simulink model "Controlador"  (R2023a)
settings: Solver=VariableStepAuto  StartTime=0.0  StopTime=60  RelTol=1e-3
values from neighbouring files (symbols this model uses):
  A = pi*R^2    (= 16971.6689129)    [Aerogerador.m]
  b = 46e3    (= 46000)    [Aerogerador.m]
  Cpmax0 = Cpmax(:, 1)    [Aerogerador.m]
  Ea_nom = Pnom/ia_nom    [Aerogerador.m]
  ia_nom = x(2, :)    [Aerogerador.m]
  J = 9e6    (= 9000000)    [Aerogerador.m]
  kv = 900*2    (= 1800)    [Aerogerador.m]
  La = 108e-3    (= 0.108)    [Aerogerador.m]
  lambdaopt = 7.5    [Aerogerador.m]    (also in funNominal.m)
  Ra = 100e-3    (= 0.1)    [Aerogerador.m]
  rho = 1.2    [Aerogerador.m]
  U_nom = x(1, :)    [Aerogerador.m]
  w_nom = (U_nom*lambdaopt)/R    [Aerogerador.m]
libraries: slpidlib x4
settings Model: Creator=danil  LastModifiedBy=danil

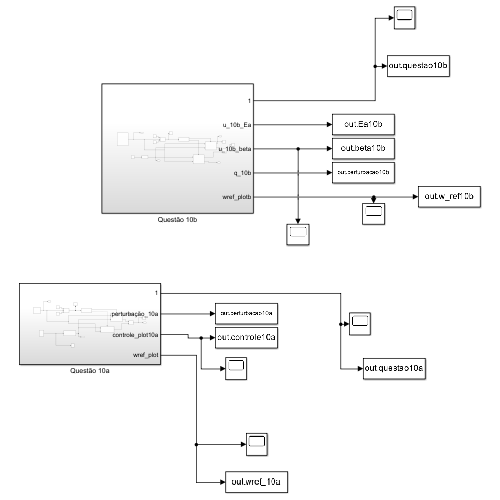
[thumbnail: Simulink's stored preview of the top-level diagram]
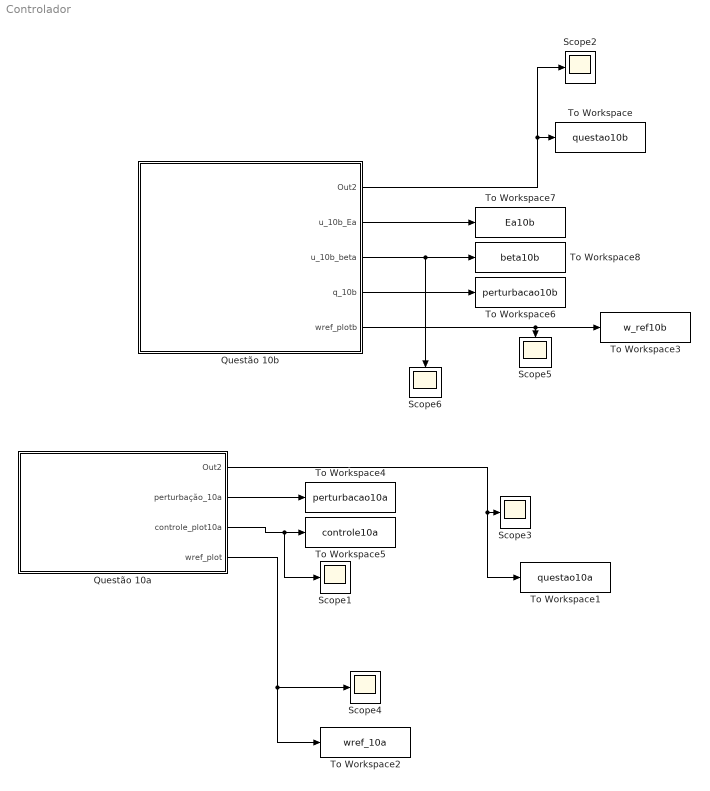
== system Controlador ==
  Questão 10a : Subsystem
  Questão 10b : Subsystem
  Scope{1..6} (6 alike) : Scope
  To Workspace : ToWorkspace  VariableName=questao10b  SampleTime=-1
      settings: Save2DSignal=2-D array (concatenate along first dimension)
  To Workspace1 : ToWorkspace  VariableName=questao10a  SampleTime=-1
      settings: Save2DSignal=2-D array (concatenate along first dimension)
  To Workspace2 : ToWorkspace  VariableName=wref_10a  SampleTime=-1
      settings: Save2DSignal=2-D array (concatenate along first dimension)
  To Workspace3 : ToWorkspace  VariableName=w_ref10b  SampleTime=-1
      settings: Save2DSignal=2-D array (concatenate along first dimension)
  To Workspace4 : ToWorkspace  VariableName=perturbacao10a  SampleTime=-1
      settings: Save2DSignal=2-D array (concatenate along first dimension)
  To Workspace5 : ToWorkspace  VariableName=controle10a  SampleTime=-1
      settings: Save2DSignal=2-D array (concatenate along first dimension)
  To Workspace6 : ToWorkspace  VariableName=perturbacao10b  SampleTime=-1
      settings: Save2DSignal=2-D array (concatenate along first dimension)
  To Workspace7 : ToWorkspace  VariableName=Ea10b  SampleTime=-1
      settings: Save2DSignal=2-D array (concatenate along first dimension)
  To Workspace8 : ToWorkspace  VariableName=beta10b  SampleTime=-1
      settings: Save2DSignal=2-D array (concatenate along first dimension)
  wires:
  Questão 10b/1(Out2) -> Scope2/1, To Workspace/1
  Questão 10a/1(Out2) -> To Workspace1/1, Scope3/1
  Questão 10a/4(wref_plot) -> To Workspace2/1, Scope4/1
  Questão 10b/5(wref_plotb) -> To Workspace3/1, Scope5/1
  Questão 10a/3(controle_plot10a) -> Scope1/1, To Workspace5/1
  Questão 10a/2(perturbação_10a) -> To Workspace4/1
  Questão 10b/4(q_10b) -> To Workspace6/1
  Questão 10b/2(u_10b_Ea) -> To Workspace7/1
  Questão 10b/3(u_10b_beta) -> Scope6/1, To Workspace8/1

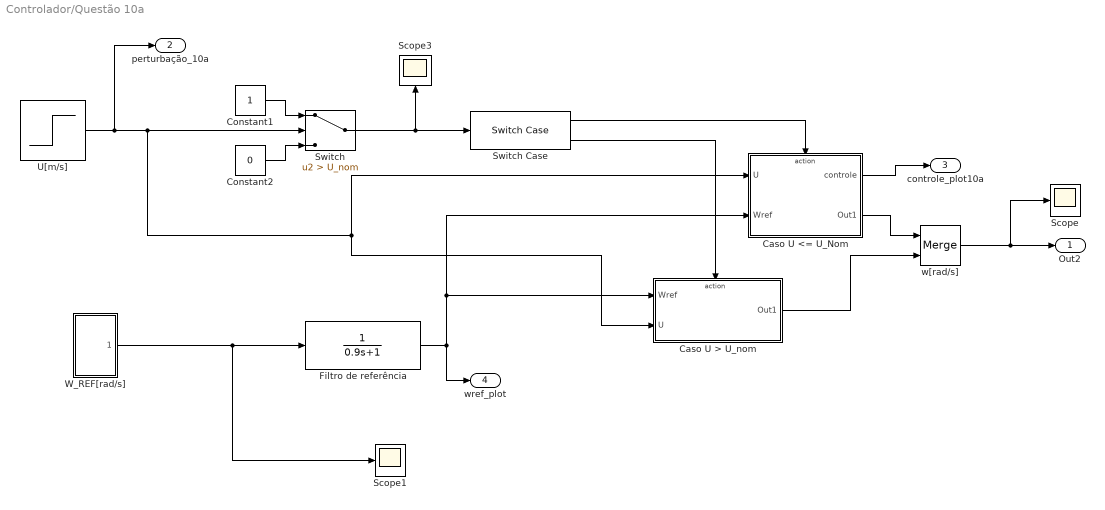
== system Controlador/Questão 10a ==
  Caso U <= U_Nom : Subsystem  TreatAsAtomicUnit=on
  Caso U > U_nom : Subsystem  TreatAsAtomicUnit=on
  Constant1 : Constant
  Constant2 : Constant  Value=0
  Filtro de referência : TransferFcn  Denominator=[0.9 1]
  Scope : Scope
  Scope1 : Scope
  Scope3 : Scope
  Switch : Switch  Criteria=u2 > Threshold  Threshold=U_nom  SaturateOnIntegerOverflow=off  InputSameDT=off
  "Switch Case " : SwitchCase  CaseConditions={0, [1]}  ShowDefaultCase=off
  U[m/s] : Step  Time=50  Before=U_nom  After=U_nom  SampleTime=0
  W_REF[rad/s] : Subsystem
  w[rad/s] : Merge
  Out2 : Outport
  perturbação_10a : Outport  Port=2
  controle_plot10a : Outport  Port=3
  wref_plot : Outport  Port=4
  wires:
  W_REF[rad/s]/1(wref_plot) -> Scope1/1, Filtro de referência/1
  U[m/s]/1 -> perturbação_10a/1, Caso U > U_nom/2(U), Caso U <= U_Nom/1(U), Switch/2
  Constant1/1 -> Switch/1
  Switch/1 -> "Switch Case "/1, Scope3/1
  Caso U > U_nom/1(Out1) -> w[rad/s]/2
  Caso U <= U_Nom/2(Out1) -> w[rad/s]/1
  Constant2/1 -> Switch/3
  w[rad/s]/1 -> Scope/1, Out2/1
  "Switch Case "/2 -> Caso U > U_nom/Action
  "Switch Case "/1 -> Caso U <= U_Nom/Action
  Caso U <= U_Nom/1(controle) -> controle_plot10a/1
  Filtro de referência/1 -> wref_plot/1, Caso U <= U_Nom/2(Wref), Caso U > U_nom/1(Wref)

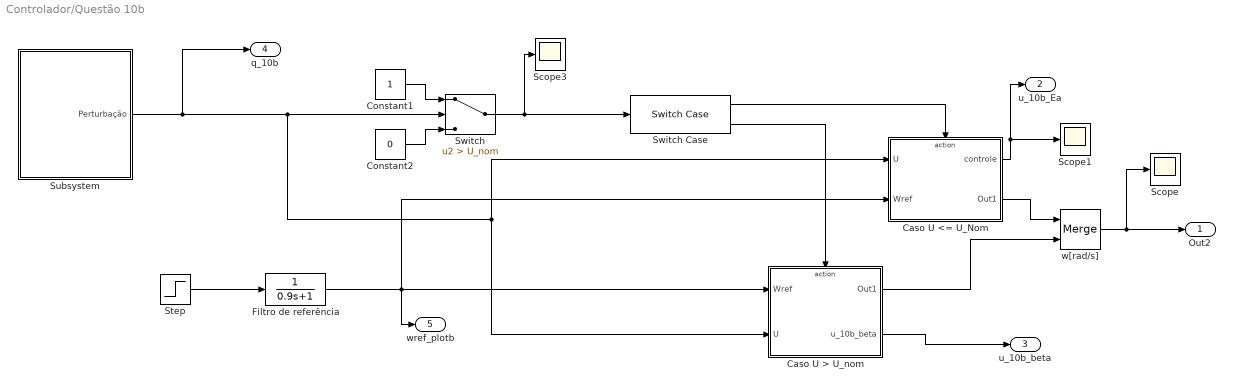
== system Controlador/Questão 10b ==
  Caso U <= U_Nom : Subsystem  TreatAsAtomicUnit=on
  Caso U > U_nom : Subsystem  TreatAsAtomicUnit=on
  Constant1 : Constant
  Constant2 : Constant  Value=0
  Filtro de referência : TransferFcn  Denominator=[0.9 1]
  Scope : Scope
  Scope1 : Scope
  Scope3 : Scope
  Step : Step  Time=10  Before=w_nom  After=w_nom  SampleTime=0
  Subsystem : Subsystem
  Switch : Switch  Criteria=u2 > Threshold  Threshold=U_nom  SaturateOnIntegerOverflow=off  InputSameDT=off
  Switch Case : SwitchCase  CaseConditions={0, [1]}  ShowDefaultCase=off
  w[rad/s] : Merge
  Out2 : Outport
  u_10b_Ea : Outport  Port=2
  u_10b_beta : Outport  Port=3
  q_10b : Outport  Port=4
  wref_plotb : Outport  Port=5
  wires:
  Caso U <= U_Nom/2(Out1) -> w[rad/s]/1
  Switch/1 -> Scope3/1, Switch Case/1
  Switch Case/1 -> Caso U <= U_Nom/Action
  Constant2/1 -> Switch/3
  Switch Case/2 -> Caso U > U_nom/Action
  Caso U > U_nom/1(Out1) -> w[rad/s]/2
  Constant1/1 -> Switch/1
  Subsystem/1(Perturbação) -> q_10b/1, Caso U > U_nom/2(U), Caso U <= U_Nom/1(U), Switch/2
  w[rad/s]/1 -> Scope/1, Out2/1
  Step/1 -> Filtro de referência/1
  Caso U <= U_Nom/1(controle) -> Scope1/1, u_10b_Ea/1
  Filtro de referência/1 -> wref_plotb/1, Caso U > U_nom/1(Wref), Caso U <= U_Nom/2(Wref)
  Caso U > U_nom/2(u_10b_beta) -> u_10b_beta/1

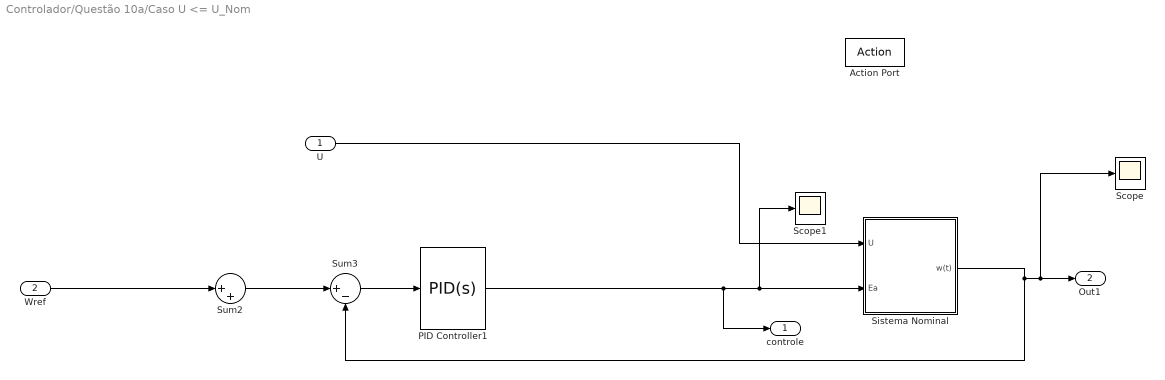
== system Controlador/Questão 10a/Caso U <= U_Nom ==
  U : Inport
  Wref : Inport  Port=2
  Action Port : ActionPort  ActionPortLabel=case [ 0 ]:
  PID Controller1 : slpidlib/PID Controller  Controller=PID  Form=Parallel  TimeDomain=Continuous-time  UseExternalTs=off  SampleTime=-1  IntegratorMethod=Forward Euler  FilterMethod=Forward Euler  ControllerParametersSource=internal  P=5586.71217162879  I=4755.74676167456  UseKiTs=off  D=1603.71676764274  N=478.091090181737  UseFilter=on  TunerSelectOption=Transfer Function Based (PID Tuner App)  InitialConditionSource=internal  InitialConditionForIntegrator=0  InitialConditionForFilter=0  DifferentiatorICPrevScaledInput=0  ExternalReset=none  TrackingMode=off  Kt=1  LimitOutput=on  SatLimitsSource=internal  UpperSaturationLimit=Ea_nom  LowerSaturationLimit=0  LinearizeAsGain=on  AntiWindupMode=none  Kb=1  LimitIntegrator=off  UpperIntegratorSaturationLimit=inf  LowerIntegratorSaturationLimit=-inf  POutMin=[]  POutMax=[]  IOutMin=[]  IOutMax=[]  DOutMin=[]  DOutMax=[]  NOutMin=[]  NOutMax=[]  SumOutMin=[]  SumOutMax=[]  SaturationOutMin=[]  SaturationOutMax=[]  PParamMin=[]  PParamMax=[]  IParamMin=[]  IParamMax=[]  DParamMin=[]  DParamMax=[]  NParamMin=[]  NParamMax=[]  KbParamMin=[]  KbParamMax=[]  KtParamMin=[]  KtParamMax=[]  KbOutMin=[]  KbOutMax=[]  KtOutMin=[]  KtOutMax=[]  IntegratorOutMin=[]  IntegratorOutMax=[]  FilterOutMin=[]  FilterOutMax=[]  SumI1OutMin=[]  SumI1OutMax=[]  SumI2OutMin=[]  SumI2OutMax=[]  SumI3OutMin=[]  SumI3OutMax=[]  SumI4OutMin=[]  SumI4OutMax=[]  SumDOutMin=[]  SumDOutMax=[]  DifferentiatorOutMin=[]  DifferentiatorOutMax=[]  FilterDiffOutCoefMin=[]  FilterDiffOutCoefMax=[]  ReciprocalOutMin=[]  ReciprocalOutMax=[]  SumDenOutMin=[]  SumDenOutMax=[]  SumNumOutMin=[]  SumNumOutMax=[]  DivideOutMin=[]  DivideOutMax=[]  UdiffTsProdOutMin=[]  UdiffTsProdOutMax=[]  NTsProdOutMin=[]  NTsProdOutMax=[]  UintegralTsProdOutMin=[]  UintegralTsProdOutMax=[]  UngainTsProdOutMin=[]  UngainTsProdOutMax=[]  ClampingZeroOutDataTypeStr=Inherit: Inherit via back propagation  ClampingZeroOutMin=[]  ClampingZeroOutMax=[]  FilterDenConstantOutDataTypeStr=Inherit: Inherit via back propagation  FilterDenConstantOutMin=[]  FilterDenConstantOutMax=[]  PCopyOutDataTypeStr=Inherit: Inherit via back propagation  PCopyOutMin=[]  PCopyOutMax=[]  NCopyOutDataTypeStr=Inherit: Inherit via back propagation  NCopyOutMin=[]  NCopyOutMax=[]  IntegratorContinuousStateAttributes=''  IntegratorStateMustResolveToSignalObject=off  IntegratorRTWStateStorageClass=Auto  FilterContinuousStateAttributes=''  FilterStateMustResolveToSignalObject=off  FilterRTWStateStorageClass=Auto  ParallelPVariant=InternalParameters  IdealPVariant=Disabled  IVariant=InternalParameters  DVariant=InternalParameters  IntegratorVariant=Continuous  SatVariant=Enabled  AWVariant=Passthrough  PCopyVariant=Disabled  TRVariant=Disabled  FdbkBlocksVariant=Forward  IdealPFdbkVariant=Disabled  SatFdbkVariant=Disabled  DerivativeFilterVariant=ContFilter  NVariant=InternalParameters  NCopyVariant=Disabled  FilterICVariant=InternalICsFilter  IntegratorICVariant=InternalICs  ExternalResetVariant=Disabled  TRSumVariant=Passthrough  SumFdbkVariant=Disabled  SumVariant=Sum_PID  TsampFilterVariant=InternalTs  TsampNgainVariant=Passthrough  TsampIntegralVariant=Disabled_SignalSpec  ExternalSaturationOutDataTypeStr=Inherit: Same as second input
  Scope : Scope
  Scope1 : Scope
  Sistema Nominal : Subsystem
  Sum2 : Sum  Inputs=|++
  Sum3 : Sum  Inputs=|+-
  controle : Outport
  Out1 : Outport  Port=2
  wires:
  U/1 -> Sistema Nominal/1(U)
  Sum3/1 -> PID Controller1/1
  Sistema Nominal/1(w(t)) -> Scope/1, Out1/1, Sum3/2
  Sum2/1 -> Sum3/1
  Wref/1 -> Sum2/1
  PID Controller1/1 -> controle/1, Scope1/1, Sistema Nominal/2(Ea)

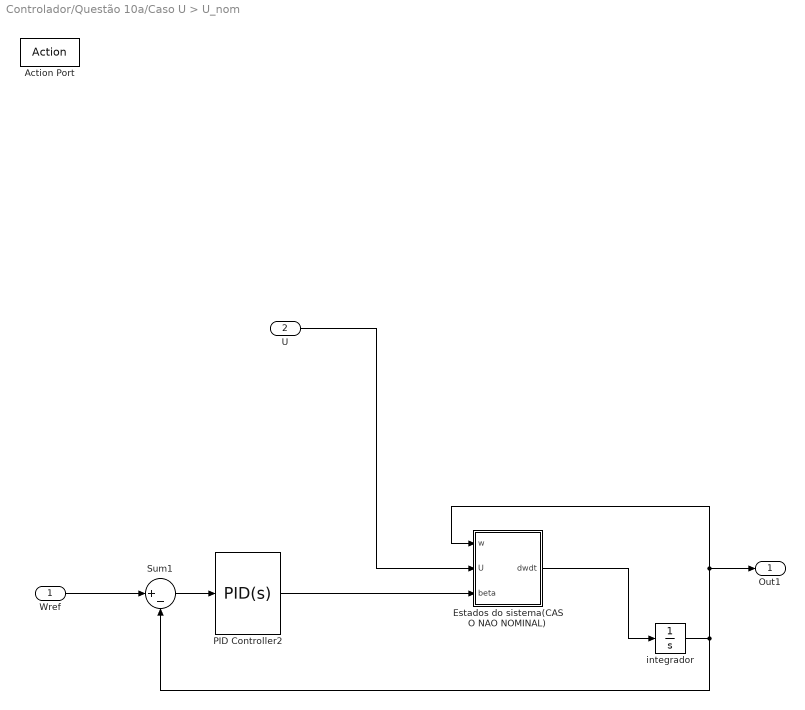
== system Controlador/Questão 10a/Caso U > U_nom ==
  Wref : Inport
  U : Inport  Port=2
  Action Port : ActionPort  ActionPortLabel=case [ 1 ]:
  Estados do sistema(CASO NAO NOMINAL) : MATLAB Function  TreatAsAtomicUnit=on
  PID Controller2 : slpidlib/PID Controller  Controller=PID  Form=Parallel  TimeDomain=Continuous-time  UseExternalTs=off  SampleTime=-1  IntegratorMethod=Forward Euler  FilterMethod=Forward Euler  ControllerParametersSource=internal  P=-0.410625599807359  I=-1.25025601800531  UseKiTs=off  D=0.00978955260280964  N=5.75949048000685  UseFilter=on  TunerSelectOption=Transfer Function Based (PID Tuner App)  InitialConditionSource=internal  InitialConditionForIntegrator=0  InitialConditionForFilter=0  DifferentiatorICPrevScaledInput=0  ExternalReset=none  TrackingMode=off  Kt=1  LimitOutput=off  SatLimitsSource=internal  UpperSaturationLimit=inf  LowerSaturationLimit=-inf  LinearizeAsGain=on  AntiWindupMode=none  Kb=1  LimitIntegrator=off  UpperIntegratorSaturationLimit=inf  LowerIntegratorSaturationLimit=-inf  POutMin=[]  POutMax=[]  IOutMin=[]  IOutMax=[]  DOutMin=[]  DOutMax=[]  NOutMin=[]  NOutMax=[]  SumOutMin=[]  SumOutMax=[]  SaturationOutMin=[]  SaturationOutMax=[]  PParamMin=[]  PParamMax=[]  IParamMin=[]  IParamMax=[]  DParamMin=[]  DParamMax=[]  NParamMin=[]  NParamMax=[]  KbParamMin=[]  KbParamMax=[]  KtParamMin=[]  KtParamMax=[]  KbOutMin=[]  KbOutMax=[]  KtOutMin=[]  KtOutMax=[]  IntegratorOutMin=[]  IntegratorOutMax=[]  FilterOutMin=[]  FilterOutMax=[]  SumI1OutMin=[]  SumI1OutMax=[]  SumI2OutMin=[]  SumI2OutMax=[]  SumI3OutMin=[]  SumI3OutMax=[]  SumI4OutMin=[]  SumI4OutMax=[]  SumDOutMin=[]  SumDOutMax=[]  DifferentiatorOutMin=[]  DifferentiatorOutMax=[]  FilterDiffOutCoefMin=[]  FilterDiffOutCoefMax=[]  ReciprocalOutMin=[]  ReciprocalOutMax=[]  SumDenOutMin=[]  SumDenOutMax=[]  SumNumOutMin=[]  SumNumOutMax=[]  DivideOutMin=[]  DivideOutMax=[]  UdiffTsProdOutMin=[]  UdiffTsProdOutMax=[]  NTsProdOutMin=[]  NTsProdOutMax=[]  UintegralTsProdOutMin=[]  UintegralTsProdOutMax=[]  UngainTsProdOutMin=[]  UngainTsProdOutMax=[]  ClampingZeroOutDataTypeStr=Inherit: Inherit via back propagation  ClampingZeroOutMin=[]  ClampingZeroOutMax=[]  FilterDenConstantOutDataTypeStr=Inherit: Inherit via back propagation  FilterDenConstantOutMin=[]  FilterDenConstantOutMax=[]  PCopyOutDataTypeStr=Inherit: Inherit via back propagation  PCopyOutMin=[]  PCopyOutMax=[]  NCopyOutDataTypeStr=Inherit: Inherit via back propagation  NCopyOutMin=[]  NCopyOutMax=[]  IntegratorContinuousStateAttributes=''  IntegratorStateMustResolveToSignalObject=off  IntegratorRTWStateStorageClass=Auto  FilterContinuousStateAttributes=''  FilterStateMustResolveToSignalObject=off  FilterRTWStateStorageClass=Auto  ParallelPVariant=InternalParameters  IdealPVariant=Disabled  IVariant=InternalParameters  DVariant=InternalParameters  IntegratorVariant=Continuous  SatVariant=Disabled  AWVariant=Passthrough  PCopyVariant=Disabled  TRVariant=Disabled  FdbkBlocksVariant=Forward  IdealPFdbkVariant=Disabled  SatFdbkVariant=Disabled  DerivativeFilterVariant=ContFilter  NVariant=InternalParameters  NCopyVariant=Disabled  FilterICVariant=InternalICsFilter  IntegratorICVariant=InternalICs  ExternalResetVariant=Disabled  TRSumVariant=Passthrough  SumFdbkVariant=Disabled  SumVariant=Sum_PID  TsampFilterVariant=InternalTs  TsampNgainVariant=Passthrough  TsampIntegralVariant=Disabled_SignalSpec  ExternalSaturationOutDataTypeStr=Inherit: Same as second input
  Sum1 : Sum  Inputs=|+-
  integrador : Integrator  InitialCondition=w_nom
  Out1 : Outport
  wires:
  Estados do sistema(CASO NAO NOMINAL)/1(dwdt) -> integrador/1
  integrador/1 -> Sum1/2, Estados do sistema(CASO NAO NOMINAL)/1(w), Out1/1
  PID Controller2/1 -> Estados do sistema(CASO NAO NOMINAL)/3(beta)
  Wref/1 -> Sum1/1
  Sum1/1 -> PID Controller2/1
  U/1 -> Estados do sistema(CASO NAO NOMINAL)/2(U)

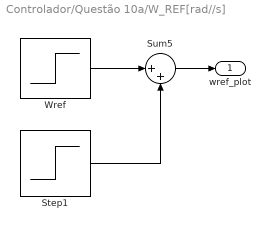
== system Controlador/Questão 10a/W_REF[rad//s] ==
  Step1 : Step  Time=40  After=w_nom/2  SampleTime=0
  Sum5 : Sum  Inputs=|++
  Wref : Step  Time=20  Before=w_nom  After=w_nom/2  SampleTime=0
  wref_plot : Outport
  wires:
  Wref/1 -> Sum5/1
  Step1/1 -> Sum5/2
  Sum5/1 -> wref_plot/1

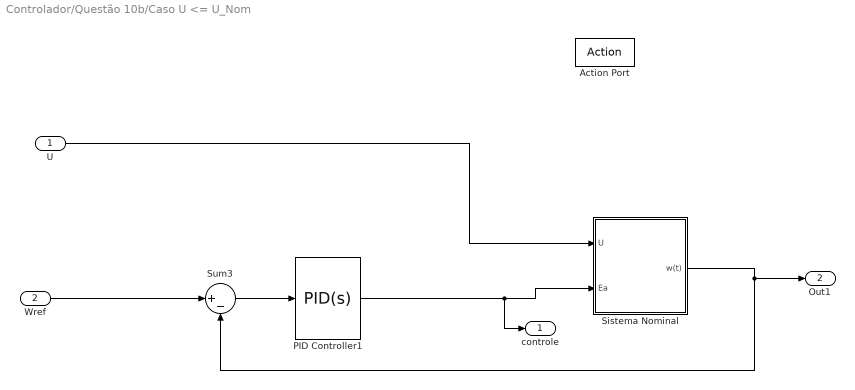
== system Controlador/Questão 10b/Caso U <= U_Nom ==
  U : Inport
  Wref : Inport  Port=2
  Action Port : ActionPort  ActionPortLabel=case [ 0 ]:
  PID Controller1 : slpidlib/PID Controller  Controller=PID  Form=Parallel  TimeDomain=Continuous-time  UseExternalTs=off  SampleTime=-1  IntegratorMethod=Forward Euler  FilterMethod=Forward Euler  ControllerParametersSource=internal  P=5586.71217162879  I=4755.74676167456  UseKiTs=off  D=1603.71676764274  N=478.091090181737  UseFilter=on  TunerSelectOption=Transfer Function Based (PID Tuner App)  InitialConditionSource=internal  InitialConditionForIntegrator=0  InitialConditionForFilter=0  DifferentiatorICPrevScaledInput=0  ExternalReset=none  TrackingMode=off  Kt=1  LimitOutput=on  SatLimitsSource=internal  UpperSaturationLimit=Ea_nom  LowerSaturationLimit=0  LinearizeAsGain=on  AntiWindupMode=none  Kb=1  LimitIntegrator=off  UpperIntegratorSaturationLimit=inf  LowerIntegratorSaturationLimit=-inf  POutMin=[]  POutMax=[]  IOutMin=[]  IOutMax=[]  DOutMin=[]  DOutMax=[]  NOutMin=[]  NOutMax=[]  SumOutMin=[]  SumOutMax=[]  SaturationOutMin=[]  SaturationOutMax=[]  PParamMin=[]  PParamMax=[]  IParamMin=[]  IParamMax=[]  DParamMin=[]  DParamMax=[]  NParamMin=[]  NParamMax=[]  KbParamMin=[]  KbParamMax=[]  KtParamMin=[]  KtParamMax=[]  KbOutMin=[]  KbOutMax=[]  KtOutMin=[]  KtOutMax=[]  IntegratorOutMin=[]  IntegratorOutMax=[]  FilterOutMin=[]  FilterOutMax=[]  SumI1OutMin=[]  SumI1OutMax=[]  SumI2OutMin=[]  SumI2OutMax=[]  SumI3OutMin=[]  SumI3OutMax=[]  SumI4OutMin=[]  SumI4OutMax=[]  SumDOutMin=[]  SumDOutMax=[]  DifferentiatorOutMin=[]  DifferentiatorOutMax=[]  FilterDiffOutCoefMin=[]  FilterDiffOutCoefMax=[]  ReciprocalOutMin=[]  ReciprocalOutMax=[]  SumDenOutMin=[]  SumDenOutMax=[]  SumNumOutMin=[]  SumNumOutMax=[]  DivideOutMin=[]  DivideOutMax=[]  UdiffTsProdOutMin=[]  UdiffTsProdOutMax=[]  NTsProdOutMin=[]  NTsProdOutMax=[]  UintegralTsProdOutMin=[]  UintegralTsProdOutMax=[]  UngainTsProdOutMin=[]  UngainTsProdOutMax=[]  ClampingZeroOutDataTypeStr=Inherit: Inherit via back propagation  ClampingZeroOutMin=[]  ClampingZeroOutMax=[]  FilterDenConstantOutDataTypeStr=Inherit: Inherit via back propagation  FilterDenConstantOutMin=[]  FilterDenConstantOutMax=[]  PCopyOutDataTypeStr=Inherit: Inherit via back propagation  PCopyOutMin=[]  PCopyOutMax=[]  NCopyOutDataTypeStr=Inherit: Inherit via back propagation  NCopyOutMin=[]  NCopyOutMax=[]  IntegratorContinuousStateAttributes=''  IntegratorStateMustResolveToSignalObject=off  IntegratorRTWStateStorageClass=Auto  FilterContinuousStateAttributes=''  FilterStateMustResolveToSignalObject=off  FilterRTWStateStorageClass=Auto  ParallelPVariant=InternalParameters  IdealPVariant=Disabled  IVariant=InternalParameters  DVariant=InternalParameters  IntegratorVariant=Continuous  SatVariant=Enabled  AWVariant=Passthrough  PCopyVariant=Disabled  TRVariant=Disabled  FdbkBlocksVariant=Forward  IdealPFdbkVariant=Disabled  SatFdbkVariant=Disabled  DerivativeFilterVariant=ContFilter  NVariant=InternalParameters  NCopyVariant=Disabled  FilterICVariant=InternalICsFilter  IntegratorICVariant=InternalICs  ExternalResetVariant=Disabled  TRSumVariant=Passthrough  SumFdbkVariant=Disabled  SumVariant=Sum_PID  TsampFilterVariant=InternalTs  TsampNgainVariant=Passthrough  TsampIntegralVariant=Disabled_SignalSpec  ExternalSaturationOutDataTypeStr=Inherit: Same as second input
  Sistema Nominal : Subsystem
  Sum3 : Sum  Inputs=|+-
  controle : Outport
  Out1 : Outport  Port=2
  wires:
  U/1 -> Sistema Nominal/1(U)
  Sum3/1 -> PID Controller1/1
  Sistema Nominal/1(w(t)) -> Out1/1, Sum3/2
  Wref/1 -> Sum3/1
  PID Controller1/1 -> controle/1, Sistema Nominal/2(Ea)

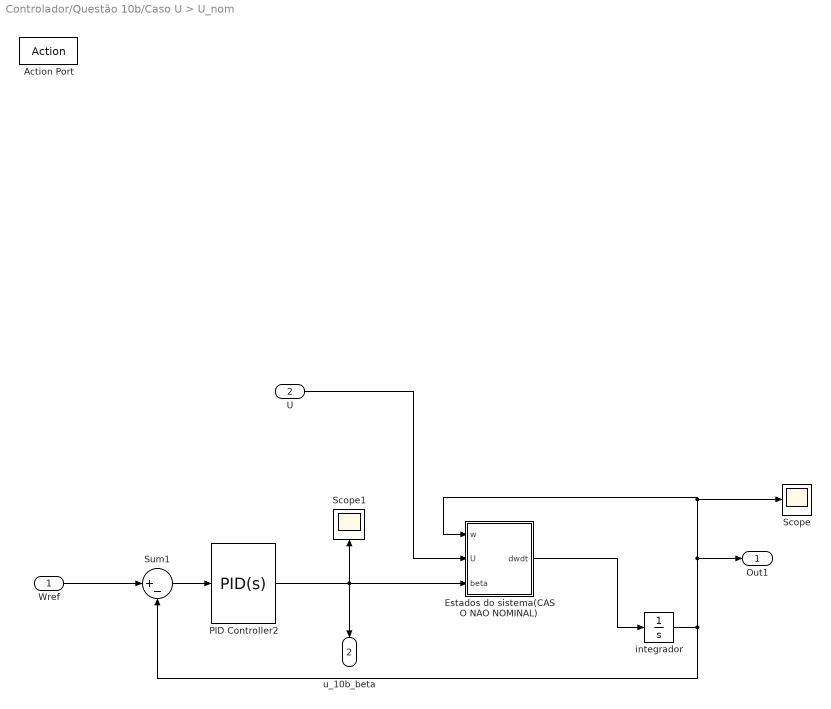
== system Controlador/Questão 10b/Caso U > U_nom ==
  Wref : Inport
  U : Inport  Port=2
  Action Port : ActionPort  ActionPortLabel=case [ 1 ]:
  Estados do sistema(CASO NAO NOMINAL) : MATLAB Function  TreatAsAtomicUnit=on
  PID Controller2 : slpidlib/PID Controller  Controller=PID  Form=Parallel  TimeDomain=Continuous-time  UseExternalTs=off  SampleTime=-1  IntegratorMethod=Forward Euler  FilterMethod=Forward Euler  ControllerParametersSource=internal  P=-0.410625599807359  I=-1.25025601800531  UseKiTs=off  D=0.00978955260280964  N=5.75949048000685  UseFilter=on  TunerSelectOption=Transfer Function Based (PID Tuner App)  InitialConditionSource=internal  InitialConditionForIntegrator=0  InitialConditionForFilter=0  DifferentiatorICPrevScaledInput=0  ExternalReset=none  TrackingMode=off  Kt=1  LimitOutput=off  SatLimitsSource=internal  UpperSaturationLimit=inf  LowerSaturationLimit=-inf  LinearizeAsGain=on  AntiWindupMode=none  Kb=1  LimitIntegrator=off  UpperIntegratorSaturationLimit=inf  LowerIntegratorSaturationLimit=-inf  POutMin=[]  POutMax=[]  IOutMin=[]  IOutMax=[]  DOutMin=[]  DOutMax=[]  NOutMin=[]  NOutMax=[]  SumOutMin=[]  SumOutMax=[]  SaturationOutMin=[]  SaturationOutMax=[]  PParamMin=[]  PParamMax=[]  IParamMin=[]  IParamMax=[]  DParamMin=[]  DParamMax=[]  NParamMin=[]  NParamMax=[]  KbParamMin=[]  KbParamMax=[]  KtParamMin=[]  KtParamMax=[]  KbOutMin=[]  KbOutMax=[]  KtOutMin=[]  KtOutMax=[]  IntegratorOutMin=[]  IntegratorOutMax=[]  FilterOutMin=[]  FilterOutMax=[]  SumI1OutMin=[]  SumI1OutMax=[]  SumI2OutMin=[]  SumI2OutMax=[]  SumI3OutMin=[]  SumI3OutMax=[]  SumI4OutMin=[]  SumI4OutMax=[]  SumDOutMin=[]  SumDOutMax=[]  DifferentiatorOutMin=[]  DifferentiatorOutMax=[]  FilterDiffOutCoefMin=[]  FilterDiffOutCoefMax=[]  ReciprocalOutMin=[]  ReciprocalOutMax=[]  SumDenOutMin=[]  SumDenOutMax=[]  SumNumOutMin=[]  SumNumOutMax=[]  DivideOutMin=[]  DivideOutMax=[]  UdiffTsProdOutMin=[]  UdiffTsProdOutMax=[]  NTsProdOutMin=[]  NTsProdOutMax=[]  UintegralTsProdOutMin=[]  UintegralTsProdOutMax=[]  UngainTsProdOutMin=[]  UngainTsProdOutMax=[]  ClampingZeroOutDataTypeStr=Inherit: Inherit via back propagation  ClampingZeroOutMin=[]  ClampingZeroOutMax=[]  FilterDenConstantOutDataTypeStr=Inherit: Inherit via back propagation  FilterDenConstantOutMin=[]  FilterDenConstantOutMax=[]  PCopyOutDataTypeStr=Inherit: Inherit via back propagation  PCopyOutMin=[]  PCopyOutMax=[]  NCopyOutDataTypeStr=Inherit: Inherit via back propagation  NCopyOutMin=[]  NCopyOutMax=[]  IntegratorContinuousStateAttributes=''  IntegratorStateMustResolveToSignalObject=off  IntegratorRTWStateStorageClass=Auto  FilterContinuousStateAttributes=''  FilterStateMustResolveToSignalObject=off  FilterRTWStateStorageClass=Auto  ParallelPVariant=InternalParameters  IdealPVariant=Disabled  IVariant=InternalParameters  DVariant=InternalParameters  IntegratorVariant=Continuous  SatVariant=Disabled  AWVariant=Passthrough  PCopyVariant=Disabled  TRVariant=Disabled  FdbkBlocksVariant=Forward  IdealPFdbkVariant=Disabled  SatFdbkVariant=Disabled  DerivativeFilterVariant=ContFilter  NVariant=InternalParameters  NCopyVariant=Disabled  FilterICVariant=InternalICsFilter  IntegratorICVariant=InternalICs  ExternalResetVariant=Disabled  TRSumVariant=Passthrough  SumFdbkVariant=Disabled  SumVariant=Sum_PID  TsampFilterVariant=InternalTs  TsampNgainVariant=Passthrough  TsampIntegralVariant=Disabled_SignalSpec  ExternalSaturationOutDataTypeStr=Inherit: Same as second input
  Scope : Scope
  Scope1 : Scope
  Sum1 : Sum  Inputs=|+-
  integrador : Integrator  InitialCondition=w_nom
  Out1 : Outport
  u_10b_beta : Outport  Port=2
  wires:
  Estados do sistema(CASO NAO NOMINAL)/1(dwdt) -> integrador/1
  integrador/1 -> Sum1/2, Estados do sistema(CASO NAO NOMINAL)/1(w), Scope/1, Out1/1
  Wref/1 -> Sum1/1
  Sum1/1 -> PID Controller2/1
  U/1 -> Estados do sistema(CASO NAO NOMINAL)/2(U)
  PID Controller2/1 -> Scope1/1, u_10b_beta/1, Estados do sistema(CASO NAO NOMINAL)/3(beta)

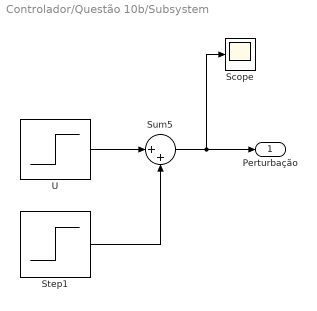
== system Controlador/Questão 10b/Subsystem ==
  Scope : Scope
  Step1 : Step  Time=40  After=-1*U_nom/2  SampleTime=0
  Sum5 : Sum  Inputs=|++
  U : Step  Time=20  Before=U_nom  After=U_nom*1.5  SampleTime=0
  Perturbação : Outport
  wires:
  U/1 -> Sum5/1
  Step1/1 -> Sum5/2
  Sum5/1 -> Scope/1, Perturbação/1

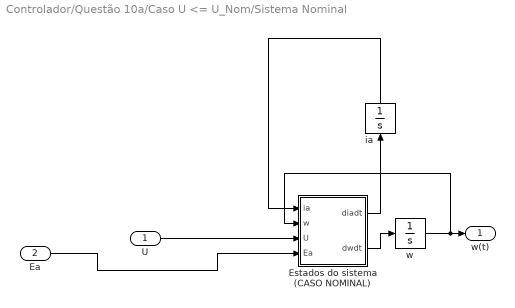
== system Controlador/Questão 10a/Caso U <= U_Nom/Sistema Nominal ==
  U : Inport
  Ea : Inport  Port=2
  Estados do sistema (CASO NOMINAL) : MATLAB Function  TreatAsAtomicUnit=on
  ia : Integrator  InitialCondition=1
  w : Integrator  InitialCondition=0.000000000000000000001
  w(t) : Outport
  wires:
  Estados do sistema (CASO NOMINAL)/2(dwdt) -> w/1
  w/1 -> Estados do sistema (CASO NOMINAL)/2(w), w(t)/1
  Estados do sistema (CASO NOMINAL)/1(diadt) -> ia/1
  ia/1 -> Estados do sistema (CASO NOMINAL)/1(ia)
  Ea/1 -> Estados do sistema (CASO NOMINAL)/4(Ea)
  U/1 -> Estados do sistema (CASO NOMINAL)/3(U)

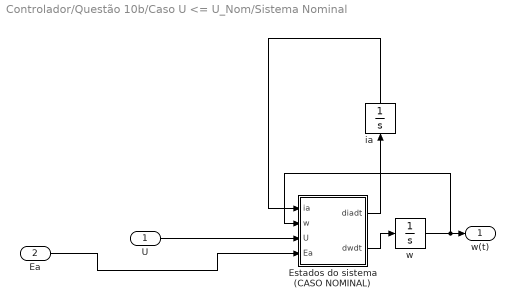
== system Controlador/Questão 10b/Caso U <= U_Nom/Sistema Nominal ==
  U : Inport
  Ea : Inport  Port=2
  Estados do sistema (CASO NOMINAL) : MATLAB Function  TreatAsAtomicUnit=on
  ia : Integrator  InitialCondition=1
  w : Integrator  InitialCondition=0.000000000000000000001
  w(t) : Outport
  wires:
  Estados do sistema (CASO NOMINAL)/2(dwdt) -> w/1
  w/1 -> Estados do sistema (CASO NOMINAL)/2(w), w(t)/1
  Estados do sistema (CASO NOMINAL)/1(diadt) -> ia/1
  ia/1 -> Estados do sistema (CASO NOMINAL)/1(ia)
  Ea/1 -> Estados do sistema (CASO NOMINAL)/4(Ea)
  U/1 -> Estados do sistema (CASO NOMINAL)/3(U)

== matlab function Controlador/Questão 10b/Caso U <= U_Nom/Sistema Nominal/Estados do sistema (CASO NOMINAL) ==
  data: ia input; w input; diadt output; dwdt output; U input; Ra parameter; J parameter; Cpmax0 parameter; A parameter; b parameter; kv parameter; La parameter; rho parameter; Ea input
function [diadt, dwdt] = fcn(ia, w, U, Ra, J, Cpmax0, A, b, kv, La, rho, Ea)



diadt = (1/La) * (kv*w - Ra*ia - Ea);
dwdt = (1/J) * ((Cpmax0*0.5*rho*A*U^3)/w - b*w - kv*ia);

== matlab function Controlador/Questão 10b/Caso U > U_nom/Estados do sistema(CASO NAO NOMINAL) ==
  data: w input; dwdt output; U input; J parameter; A parameter; b parameter; kv parameter; rho parameter; ia_nom parameter; beta input; lambdaopt parameter
function dwdt  = fcn(w, U, J, A, b, kv, rho, ia_nom, beta, lambdaopt)


Cp = (0.44 - 0.167*beta)*sin((pi*lambdaopt)/(15 - 0.3*beta)) - 0.16*lambdaopt*beta;

dwdt = (1/J) * ((Cp*0.5*rho*A*U^3)/w - b*w - kv*ia_nom);

== matlab function Controlador/Questão 10a/Caso U <= U_Nom/Sistema Nominal/Estados do sistema (CASO NOMINAL) ==
  data: ia input; w input; diadt output; dwdt output; U input; Ra parameter; J parameter; Cpmax0 parameter; A parameter; b parameter; kv parameter; La parameter; rho parameter; Ea input
function [diadt, dwdt] = fcn(ia, w, U, Ra, J, Cpmax0, A, b, kv, La, rho, Ea)



diadt = (1/La) * (kv*w - Ra*ia - Ea);
dwdt = (1/J) * ((Cpmax0*0.5*rho*A*U^3)/w - b*w - kv*ia);

== matlab function Controlador/Questão 10a/Caso U > U_nom/Estados do sistema(CASO NAO NOMINAL) ==
  data: w input; dwdt output; U input; J parameter; A parameter; b parameter; kv parameter; rho parameter; ia_nom parameter; beta input; lambdaopt parameter
function dwdt  = fcn(w, U, J, A, b, kv, rho, ia_nom, beta, lambdaopt)


Cp = (0.44 - 0.167*beta)*sin((pi*lambdaopt)/(15 - 0.3*beta)) - 0.16*lambdaopt*beta;

dwdt = (1/J) * ((Cp*0.5*rho*A*U^3)/w - b*w - kv*ia_nom);
